simulink model "fm_gram"  (R2025b)
settings: Solver=ode2  StartTime=0.0  StopTime=5  FixedStep=1/400  RelTol=1e-3  EnableMultiTasking=on
PreLoadFcn:
  | stepsize_fm = evalin('base', get_param(bdroot, 'FixedStep'));
undefined symbols (not defined in the file or in its folder): Earth, F, Light, magnitude, MIL, propulsion, servo, vehicle, WGS84
libraries: slrealtimeutilitieslib x4, aerolibwind2 x2, sharedtransform x1, aerolib6dof2 x1, aerolibatmos2 x1, aerolibobsolete x1, slrealtimeiplib x1
settings Model: Creator=ac112430  LastModifiedBy=ac124458
settings SolverCC: AlgebraicLoopSolver=LineSearch
settings DataIOCC: ReturnWorkspaceOutputs=off
settings OptimizationCC: LifeSpan=inf
settings DebuggingCC: UnconnectedInputMsg=warning  UnconnectedOutputMsg=warning  UnconnectedLineMsg=warning  SFUnexpectedBacktrackingDiag=warning  SFNoUnconditionalDefaultTransitionDiag=warning  SFExecutionAtInitializationDiag=none  ArithmeticOperatorsInVariantConditions=warning
settings ModelReferenceCC: EnableRefExpFcnMdlSchedulingChecks=on
settings SFSimCC: SimUseLocalCustomCode=off  CustomCodeUndefinedFunction=UseInterfaceOnly
settings RTWCC: RTWUseLocalCustomCode=off  GPUComputeCapability=3.5
settings CodeAppCC: StateflowObjectComments=on
settings GRTTargetCC: TargetLangStandard=C89/C90 (ANSI)
settings ConfigComp: CovMetricSettings=dw  CovSaveCumulativeToWorkspaceVar=on  CovSaveSingleToWorkspaceVar=on  CovExternalEMLEnable=off

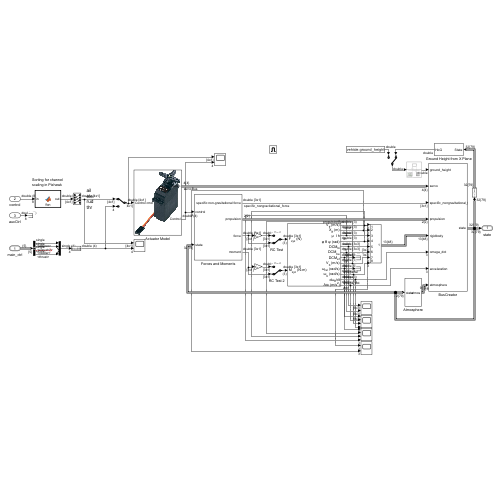
[thumbnail: Simulink's stored preview of the top-level diagram]
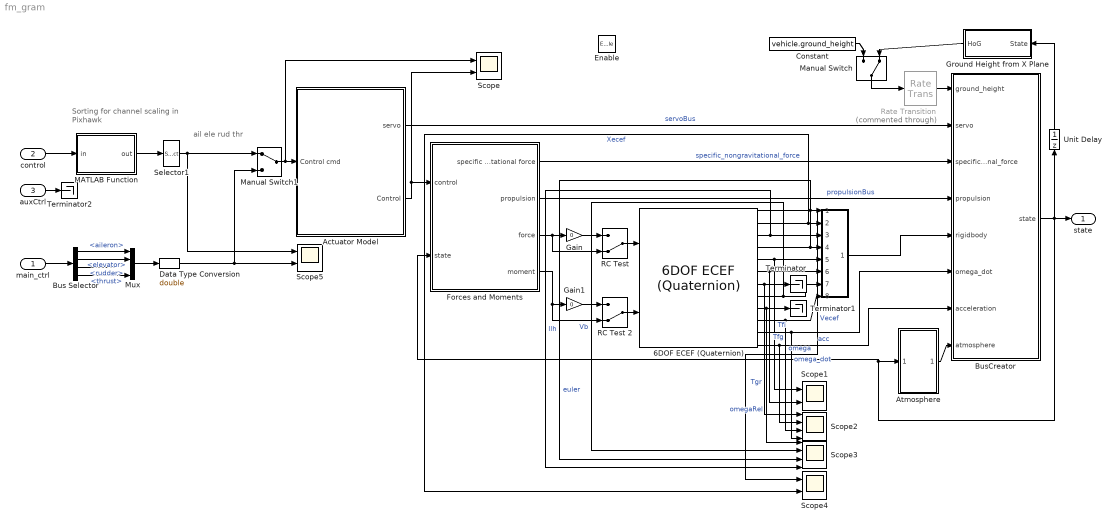
== system fm_gram ==
  note: ail
      | ele
      | rud
      | thr
  note: Sorting for channel
      | scaling in Pixhawk
  main_ctrl : Inport  OutDataTypeStr=Bus: main_ctrl_axes_bus  PortDimensions=1
  control : Inport  Port=2  PortDimensions=8
  auxCtrl : Inport  Port=3  PortDimensions=8
  Enable : EnablePort  PropagateVarSize=During execution
  " " : Subsystem
  6DOF ECEF (Quaternion) : aerolib6dof2/6DOF ECEF (Quaternion)  units=Metric (MKS)  mtype=Fixed  xg_0=vehicle.pos0  Vm_0=vehicle.vel0  eul_0=vehicle.ori0  pm_0=vehicle.omega0  mass_0=vehicle.m  mass_e=0.5  mass_f=2.0  inertia=vehicle.J  inertia_e=eye(3)  inertia_f=2*eye(3)  vre_flag=on  abi_flag=off  ptype=Earth (WGS84)  R=6378137  F=1/298.257223563  w_E=7292115e-11  angle_in=Internal  LPM0=0  quat_statename=''  pm_statename=''  Vm_statename=''  posfixedframe_statename=''  posinertial_statename=''  LPM_statename=''  mass_statename=''
  Actuator Model : Subsystem
      mask Display: image('figures\servo.jpg');
  Atmosphere : Subsystem
  Bus Selector : BusSelector  OutputSignals=aileron,elevator,rudder,thrust
  BusCreator : Subsystem
  Constant : Constant  Value=vehicle.ground_height  SampleTime=stepsize_fm
  Data Type Conversion : DataTypeConversion  OutDataTypeStr=double  SaturateOnIntegerOverflow=off  RndMeth=Floor
  Forces and Moments : Subsystem
  Gain : Gain  Gain=0
  Gain1 : Gain  Gain=0
  Ground Height from X Plane : Subsystem
  MATLAB Function : MATLAB Function  TreatAsAtomicUnit=on
  Manual Switch : ManualSwitch  CurrentSetting=0
  Manual Switch1 : ManualSwitch
  Mux : Mux
  RC Test : ManualSwitch  CurrentSetting=0
  RC Test 2 : ManualSwitch  CurrentSetting=0
  Rate Transition : RateTransition  Commented=through
  Scope{,1,4..5} (4 alike) : Scope  NumInputPorts=2
      Scope settings: ActiveDisplayYMinimum=-1.25  ActiveDisplayYMaximum=1.25
      Scope1 settings: ActiveDisplayYMinimum=-1  ActiveDisplayYMaximum=1  DataLoggingVariableName=ScopeData6
      Scope4 settings: ActiveDisplayYMinimum=-1.2221205757551141  ActiveDisplayYMaximum=1.2469022861950132  DataLoggingVariableName=ScopeData9
      Scope5 settings: ActiveDisplayYMinimum=-1.2414850783724674  ActiveDisplayYMaximum=1.2585150520126931
  Scope2 : Scope  NumInputPorts=4
      settings: ActiveDisplayYMinimum=-1  ActiveDisplayYMaximum=1  DataLoggingVariableName=ScopeData7
  Scope3 : Scope  NumInputPorts=4
      settings: ActiveDisplayYMinimum=-21.853179685501779  ActiveDisplayYMaximum=14.273381039110083  DataLoggingVariableName=ScopeData8
  Selector1 : Selector  InputPortWidth=4  IndexOptions=Index vector (dialog)  Indices=[2 3 4 1]  OutputSizes=1  RuntimeRangeChecks=on
  Terminator : Terminator
  Terminator1 : Terminator
  Terminator2 : Terminator
  Unit Delay : UnitDelay  SampleTime=-1  HasFrameUpgradeWarning=on
  state : Outport  OutDataTypeStr=Bus: fmBus  VectorParamsAs1DForOutWhenUnconnected=off
  wires:
  Forces and Moments/1(specific non-gravitational force) -> BusCreator/3(specific_nongravitational_force)  "specific_nongravitational_force"
  6DOF ECEF (Quaternion)/3 -> Scope3/4, " "/3(In3)  "llh"
  6DOF ECEF (Quaternion)/6 -> Scope1/2, " "/6(In6)  "Tfg"
  6DOF ECEF (Quaternion)/5 -> Scope1/1, " "/5(In5)  "Tfi"
  6DOF ECEF (Quaternion)/2 -> Scope4/2, " "/2(In2)  "Xecef"
  6DOF ECEF (Quaternion)/1 -> Scope4/1, " "/1(In1)  "Vecef"
  6DOF ECEF (Quaternion)/12 -> Scope2/2, BusCreator/7(acceleration)  "acc"
  6DOF ECEF (Quaternion)/8 -> Scope3/2, " "/7(In8)  "Vb"
  6DOF ECEF (Quaternion)/11 -> Scope2/4, BusCreator/6(omega_dot)  "omega_dot"
  Forces and Moments/2(propulsion) -> BusCreator/4(propulsion)  "propulsionBus"
  6DOF ECEF (Quaternion)/7 -> Scope2/1, Terminator/1  "Tgr"
  6DOF ECEF (Quaternion)/9 -> Terminator1/1, Scope3/1  "omegaRel"
  6DOF ECEF (Quaternion)/10 -> Scope2/3, " "/8(In10)  "omega"
  6DOF ECEF (Quaternion)/4 -> Scope3/3, " "/4(In4)  "euler"
  " "/1(Out1) -> BusCreator/5(rigidbody)
  Gain/1 -> RC Test/1
  Forces and Moments/3(force) -> RC Test/2, Gain/1
  Gain1/1 -> RC Test 2/1
  Forces and Moments/4(moment) -> RC Test 2/2, Gain1/1
  Actuator Model/2(Control) -> Scope/2, Forces and Moments/1(control)
  MATLAB Function/1(out) -> Selector1/1
  Actuator Model/1(servo) -> BusCreator/2(servo)  "servoBus"
  Ground Height from X Plane/1(HoG) -> Manual Switch/2
  Rate Transition/1 -> BusCreator/1(ground_height)
  control/1 -> MATLAB Function/1(in)
  Unit Delay/1 -> Ground Height from X Plane/1(State)
  auxCtrl/1 -> Terminator2/1
  Manual Switch/1 -> Rate Transition/1
  Constant/1 -> Manual Switch/1
  BusCreator/1(state) -> Forces and Moments/2(state), Atmosphere/1(state), Unit Delay/1, state/1
  Atmosphere/1(atmos) -> BusCreator/8(atmosphere)
  RC Test/1 -> 6DOF ECEF (Quaternion)/1
  RC Test 2/1 -> 6DOF ECEF (Quaternion)/2
  Mux/1 -> Data Type Conversion/1
  main_ctrl/1 -> Bus Selector/1
  Bus Selector/1 -> Mux/1  "<aileron>"
  Bus Selector/2 -> Mux/2  "<elevator>"
  Bus Selector/3 -> ?  "<rudder>"
  Bus Selector/4 -> Mux/4  "<thrust>"
  Selector1/1 -> Scope5/1, Manual Switch1/1
  Data Type Conversion/1 -> Manual Switch1/2, Scope5/2
  Manual Switch1/1 -> Scope/1, Actuator Model/1(Control cmd)

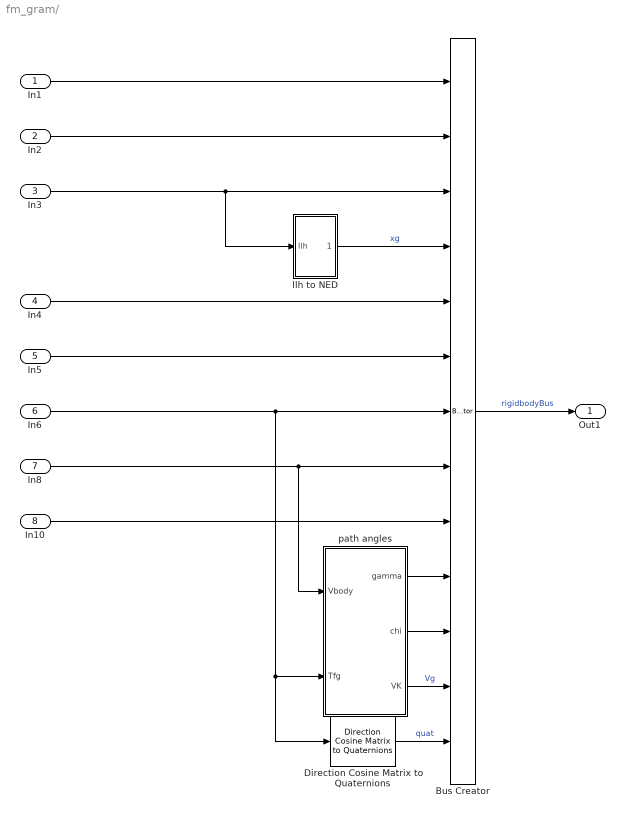
== system fm_gram/  ==
  In1 : Inport
  In2 : Inport  Port=2
  In3 : Inport  Port=3
  In4 : Inport  Port=4
  In5 : Inport  Port=5
  In6 : Inport  Port=6
  In8 : Inport  Port=7
  In10 : Inport  Port=8
  Bus Creator : BusCreator  Inputs=13  OutDataTypeStr=Bus: rigidbodyBus
  Direction Cosine Matrix to Quaternions : sharedtransform/Direction Cosine Matrix  to Quaternions  aMode=aMode  action=None  tolerance=eps(2)
  llh to NED : Subsystem
  path angles : MATLAB Function  TreatAsAtomicUnit=on
  Out1 : Outport  VectorParamsAs1DForOutWhenUnconnected=off
  wires:
  In10/1 -> Bus Creator/9
  path angles/2(chi) -> Bus Creator/11
  path angles/1(gamma) -> Bus Creator/10
  Direction Cosine Matrix to Quaternions/1 -> Bus Creator/13  "quat"
  In1/1 -> Bus Creator/1
  path angles/3(VK) -> Bus Creator/12  "Vg"
  In3/1 -> llh to NED/1(llh), Bus Creator/3
  In2/1 -> Bus Creator/2
  Bus Creator/1 -> Out1/1  "rigidbodyBus"
  In4/1 -> Bus Creator/5
  In8/1 -> path angles/1(Vbody), Bus Creator/8
  In6/1 -> Bus Creator/7, path angles/2(Tfg), Direction Cosine Matrix to Quaternions/1
  In5/1 -> Bus Creator/6
  llh to NED/1(NED) -> Bus Creator/4  "xg"

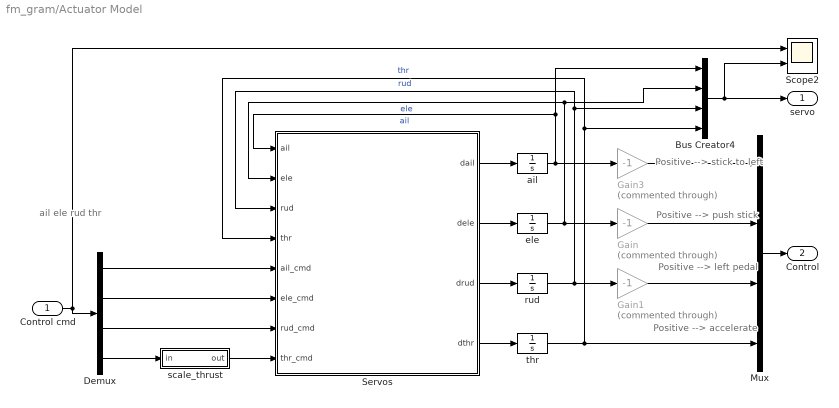
== system fm_gram/Actuator Model ==
  note: ail
      | ele
      | rud
      | thr
  note: Positive --> stick to left
  note: Positive --> left pedal
  note: Positive --> accelerate
  note: Positive --> push stick
  Control cmd : Inport
  Bus Creator4 : BusCreator  Inputs=4  OutDataTypeStr=Bus: servoBus
  Demux : Demux
  Gain : Gain  Commented=through  Gain=-1
  Gain1 : Gain  Commented=through  Gain=-1
  Gain3 : Gain  Commented=through  Gain=-1
  Mux : Mux
  Scope2 : Scope  NumInputPorts=2
      settings: ActiveDisplayYMinimum=-1.125  ActiveDisplayYMaximum=0.12499999999999997
  Servos : MATLAB Function  TreatAsAtomicUnit=on
  ail : Integrator  LimitOutput=on  UpperSaturationLimit=servo.ailLim(1)  LowerSaturationLimit=servo.ailLim(2)
  ele : Integrator  LimitOutput=on  UpperSaturationLimit=servo.eleLim(1)  LowerSaturationLimit=servo.eleLim(2)
  rud : Integrator  LimitOutput=on  UpperSaturationLimit=servo.rudLim(1)  LowerSaturationLimit=servo.rudLim(2)
  scale_thrust : MATLAB Function  TreatAsAtomicUnit=on
  thr : Integrator  LimitOutput=on  UpperSaturationLimit=servo.deltLim(1)  LowerSaturationLimit=servo.deltLim(2)
  servo : Outport  OutDataTypeStr=Bus: servoBus  VectorParamsAs1DForOutWhenUnconnected=off
  Control : Outport  Port=2
  wires:
  thr/1 -> Servos/4(thr), Bus Creator4/4, Mux/4  "thr"
  rud/1 -> Servos/3(rud), Bus Creator4/3, Gain1/1  "rud"
  ele/1 -> Bus Creator4/2, Servos/2(ele), Gain/1  "ele"
  Servos/4(dthr) -> thr/1
  Servos/1(dail) -> ail/1
  ail/1 -> Bus Creator4/1, Servos/1(ail), Gain3/1  "ail"
  Bus Creator4/1 -> Scope2/2, servo/1
  Control cmd/1 -> Scope2/1, Demux/1
  Mux/1 -> Control/1
  Demux/4 -> scale_thrust/1(in)
  Demux/3 -> Servos/7(rud_cmd)
  Demux/2 -> Servos/6(ele_cmd)
  Demux/1 -> Servos/5(ail_cmd)
  Servos/2(dele) -> ele/1
  Servos/3(drud) -> rud/1
  Gain/1 -> Mux/2
  Gain1/1 -> Mux/3
  Gain3/1 -> Mux/1
  scale_thrust/1(out) -> Servos/8(thr_cmd)

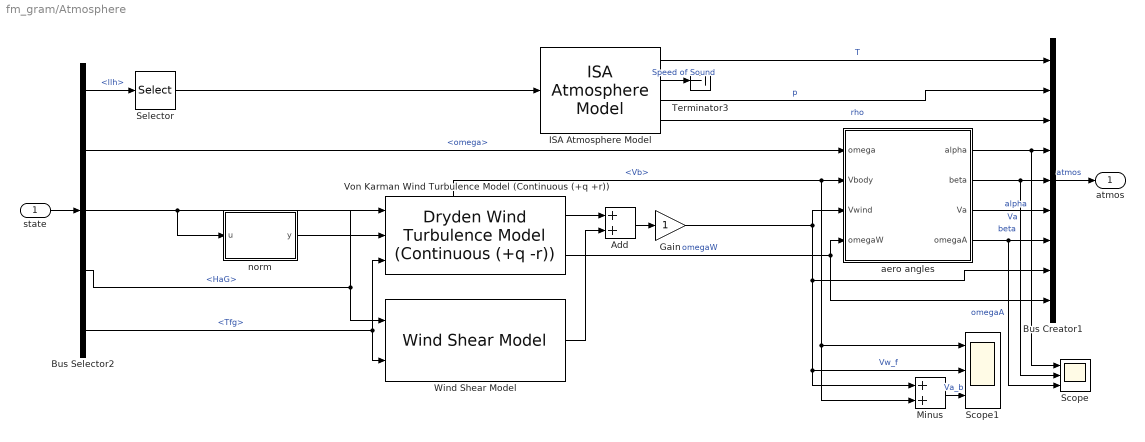
== system fm_gram/Atmosphere ==
  state : Inport
  Add : Sum
  Bus Creator1 : BusCreator  Inputs=9  OutDataTypeStr=Bus: atmosBus
  Bus Selector2 : BusSelector  OutputSignals=rigidbodyBus.llh,rigidbodyBus.omega,rigidbodyBus.Vb,utilityBus.HaG,rigidbodyBus.Tfg
  Gain : Gain
  ISA Atmosphere Model : aerolibatmos2/ISA Atmosphere Model  useExtended=off  action=None  custom=off  viscosityOut=off  g=9.80665  gamma=1.4  R=287.0531  L=0.0065  h_trop=11000  h_strat=20000  rho0=1.225  P0=101325  T0=288.15  h0=0  S=110.4  Tref=273.15  muref=1.716e-5
  Minus : Sum
  Scope : Scope  NumInputPorts=3
      settings: ActiveDisplayYMinimum=-2.50048  ActiveDisplayYMaximum=2.33546  DataLoggingVariableName=ScopeData3
  Scope1 : Scope  NumInputPorts=3
      settings: ActiveDisplayYMinimum=-12.555961798093179  ActiveDisplayYMaximum=23.617329088677021
  Selector : Selector  InputPortWidth=3  IndexOptions=Index vector (dialog)  Indices=3  OutputSizes=1
  Terminator3 : Terminator
  Von Karman Wind Turbulence Model (Continuous (+q +r)) : aerolibwind2/Dryden Wind Turbulence Model  (Continuous (+q -r))  units=Metric (MKS)  spec=MIL-F-8785C  model=Continuous Von Karman (+q +r)  W20=atmosphere.windStrength  Wdeg=atmosphere.windDir  TurbProb=10^-2 - Light  L_high=410  Wingspan=aerodynamic.b  ts=stepsize_fm  Seed=randi(20000,1,4)  T_on=off
  Wind Shear Model : aerolibwind2/Wind Shear Model  units=Metric (MKS)  phase=Other  W_20=atmosphere.windStrength  Wdeg=atmosphere.windDir
  aero angles : MATLAB Function  TreatAsAtomicUnit=on
  norm : MATLAB Function  TreatAsAtomicUnit=on
  atmos : Outport  OutDataTypeStr=Bus: atmosBus  VectorParamsAs1DForOutWhenUnconnected=off
  wires:
  Bus Creator1/1 -> atmos/1  "atmos"
  ISA Atmosphere Model/3 -> Bus Creator1/2  "p"
  ISA Atmosphere Model/1 -> Bus Creator1/1  "T"
  ISA Atmosphere Model/2 -> Terminator3/1  "Speed of Sound"
  Bus Selector2/1 -> Selector/1  "<llh>"
  Selector/1 -> ISA Atmosphere Model/1
  ISA Atmosphere Model/4 -> Bus Creator1/3  "rho"
  aero angles/1(alpha) -> Scope/1, Bus Creator1/4  "alpha"
  aero angles/2(beta) -> Scope/2, Bus Creator1/5  "beta"
  state/1 -> Bus Selector2/1
  Bus Selector2/2 -> aero angles/1(omega)  "<omega>"
  Wind Shear Model/1 -> Add/2
  norm/1(y) -> Von Karman Wind Turbulence Model (Continuous (+q +r))/2
  Von Karman Wind Turbulence Model (Continuous (+q +r))/1 -> Add/1
  Von Karman Wind Turbulence Model (Continuous (+q +r))/2 -> Bus Creator1/9, aero angles/4(omegaW)  "omegaW"
  Add/1 -> Gain/1
  Bus Selector2/5 -> Wind Shear Model/2, Von Karman Wind Turbulence Model (Continuous (+q +r))/3  "<Tfg>"
  aero angles/4(omegaA) -> Bus Creator1/7, Scope/3  "omegaA"
  Bus Selector2/4 -> Von Karman Wind Turbulence Model (Continuous (+q +r))/1, Wind Shear Model/1  "<HaG>"
  aero angles/3(Va) -> Bus Creator1/6  "Va"
  Minus/1 -> Scope1/3  "Va_b"
  Bus Selector2/3 -> Minus/2, Scope1/1, aero angles/2(Vbody), norm/1(u)  "<Vb>"
  Gain/1 -> Bus Creator1/8, Scope1/2, Minus/1, aero angles/3(Vwind)  "Vw_f"

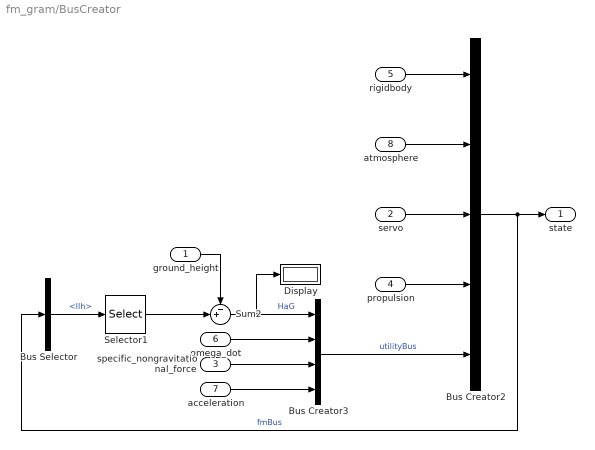
== system fm_gram/BusCreator ==
  ground_height : Inport
  servo : Inport  Port=2  OutDataTypeStr=Bus: servoBus
  specific_nongravitational_force : Inport  Port=3
  propulsion : Inport  Port=4  OutDataTypeStr=Bus: propulsionBus
  rigidbody : Inport  Port=5  OutDataTypeStr=Bus: rigidbodyBus
  omega_dot : Inport  Port=6
  acceleration : Inport  Port=7
  atmosphere : Inport  Port=8  OutDataTypeStr=Bus: atmosBus
  Bus Creator2 : BusCreator  Inputs=5  OutDataTypeStr=Bus: fmBus
  Bus Creator3 : BusCreator  Inputs=4  OutDataTypeStr=Bus: utilityBus
  Bus Selector : BusSelector  OutputSignals=rigidbodyBus.llh
  Display : Display
  Selector1 : Selector  InputPortWidth=3  IndexOptions=Index vector (dialog)  Indices=3  OutputSizes=1
  Sum2 : Sum  Inputs=-+|
  state : Outport  OutDataTypeStr=Bus: fmBus  VectorParamsAs1DForOutWhenUnconnected=off
  wires:
  Sum2/1 -> Display/1, Bus Creator3/1  "HaG"
  propulsion/1 -> Bus Creator2/4
  servo/1 -> Bus Creator2/3
  Bus Creator3/1 -> Bus Creator2/5  "utilityBus"
  Bus Creator2/1 -> state/1, Bus Selector/1  "fmBus"
  atmosphere/1 -> Bus Creator2/2
  Bus Selector/1 -> Selector1/1  "<llh>"
  rigidbody/1 -> Bus Creator2/1
  specific_nongravitational_force/1 -> Bus Creator3/3
  Selector1/1 -> Sum2/2
  ground_height/1 -> Sum2/1
  omega_dot/1 -> Bus Creator3/2
  acceleration/1 -> Bus Creator3/4

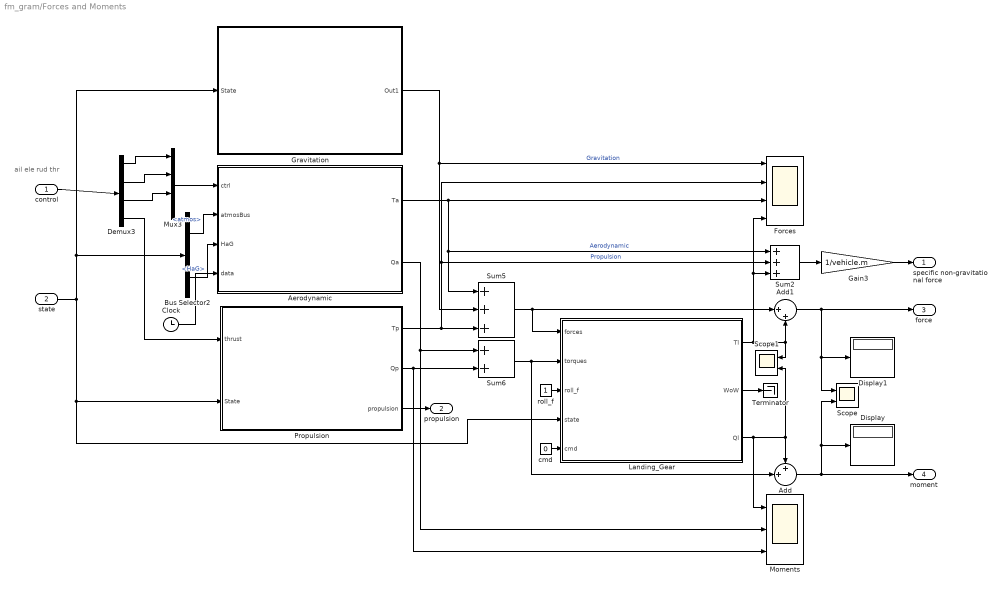
== system fm_gram/Forces and Moments ==
  note: ail
      | ele
      | rud
      | thr
  control : Inport
  state : Inport  Port=2
  Add : Sum  Inputs=++|
  Add1 : Sum  Inputs=|++
  Aerodynamic : MATLAB Function  TreatAsAtomicUnit=on
  Bus Selector2 : BusSelector  OutputSignals=atmos,utilityBus.HaG
  Clock : Clock
  Demux3 : Demux
  Display : Display
  Display1 : Display
  Forces : Scope  NumInputPorts=4
      settings: ActiveDisplayYMinimum=-8.4836089188338661  ActiveDisplayYMaximum=44.535465531132829
  Gain3 : Gain  Gain=1/vehicle.m
  Gravitation : Subsystem
      mask Display: image('figures\gravitation.jpg');
  Landing_Gear : Subsystem
      mask Display: image('C:\Workspace\funcub-xl\figures\LG.jpg'); % Use "Edit Image" on toolstrip to change.
  Moments : Scope  NumInputPorts=3
      settings: ActiveDisplayYMinimum=-12.453646898269653  ActiveDisplayYMaximum=7.4078247547149658  DataLoggingVariableName=ScopeData2
  Mux3 : Mux
  Propulsion : Subsystem
      mask Display: image('figures\propulsion.jpg');
  Scope : Scope  NumInputPorts=2
      settings: ActiveDisplayYMinimum=-87.1188785359822  ActiveDisplayYMaximum=56.206165438850242
  Scope1 : Scope  NumInputPorts=2
      settings: ActiveDisplayYMinimum=-7.91236  ActiveDisplayYMaximum=9.60283
  Sum2 : Sum  Inputs=+++
  Sum5 : Sum  Inputs=+++
  Sum6 : Sum
  Terminator : Terminator
  cmd : Constant  Value=0
  roll_f : Constant
  specific non-gravitational force : Outport  VectorParamsAs1DForOutWhenUnconnected=off
  propulsion : Outport  Port=2  VectorParamsAs1DForOutWhenUnconnected=off
  force : Outport  Port=3  VectorParamsAs1DForOutWhenUnconnected=off
  moment : Outport  Port=4  VectorParamsAs1DForOutWhenUnconnected=off
  wires:
  Gain3/1 -> specific non-gravitational force/1
  Demux3/4 -> Propulsion/1(thrust)
  control/1 -> Demux3/1
  Propulsion/3(propulsion) -> propulsion/1
  Gravitation/1(Out1) -> Sum5/2, Forces/1  "Gravitation"
  Demux3/2 -> Mux3/2
  Demux3/3 -> Mux3/3
  Demux3/1 -> Mux3/1
  Aerodynamic/1(Ta) -> Forces/3, Sum5/1, Sum2/1  "Aerodynamic"
  Propulsion/1(Tp) -> Forces/2, Sum2/2, Sum5/3  "Propulsion"
  roll_f/1 -> Landing_Gear/3(roll_f)
  Landing_Gear/1(Tl) -> Add1/2, Scope1/1, Forces/4, Sum2/3
  Landing_Gear/3(Ql) -> Moments/1, Scope1/2, Add/1
  state/1 -> Landing_Gear/4(state), Propulsion/2(State), Gravitation/1(State), Bus Selector2/1
  Bus Selector2/1 -> Aerodynamic/2(atmosBus)  "<atmos>"
  Bus Selector2/2 -> Aerodynamic/3(HaG)  "<HaG>"
  Mux3/1 -> Aerodynamic/1(ctrl)
  Add1/1 -> Display1/1, Scope/1, force/1
  Add/1 -> moment/1, Scope/2, Display/1
  Sum2/1 -> Gain3/1
  Propulsion/2(Qp) -> Moments/3, Sum6/2
  Aerodynamic/2(Qa) -> Moments/2, Sum6/1
  Sum5/1 -> Add1/1, Landing_Gear/1(forces)
  Sum6/1 -> Add/2, Landing_Gear/2(torques)
  Landing_Gear/2(WoW) -> Terminator/1
  Clock/1 -> Aerodynamic/4(data)
  cmd/1 -> Landing_Gear/5(cmd)

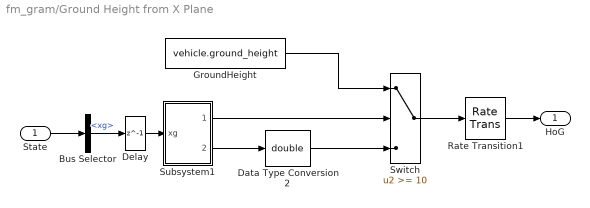
== system fm_gram/Ground Height from X Plane ==
  State : Inport
  Bus Selector : BusSelector  OutputSignals=rigidbodyBus.xg
  Data Type Conversion2 : DataTypeConversion  OutDataTypeStr=double  SaturateOnIntegerOverflow=off  RndMeth=Floor
  Delay : Delay  DelayLength=1
  GroundHeight : Constant  Value=vehicle.ground_height  SampleTime=-1
  Rate Transition1 : RateTransition  OutPortSampleTime=stepsize_fm
  Subsystem1 : Subsystem
  Switch : Switch  Threshold=10  SaturateOnIntegerOverflow=off  InputSameDT=off
  HoG : Outport  VectorParamsAs1DForOutWhenUnconnected=off
  wires:
  Subsystem1/2(Out1) -> Data Type Conversion2/1
  Rate Transition1/1 -> HoG/1
  Switch/1 -> Rate Transition1/1
  GroundHeight/1 -> Switch/1
  Data Type Conversion2/1 -> Switch/3
  Subsystem1/1(Out2) -> Switch/2
  Delay/1 -> Subsystem1/1(xg)
  State/1 -> Bus Selector/1
  Bus Selector/1 -> Delay/1  "<xg>"

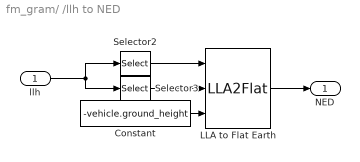
== system fm_gram/ /llh to NED ==
  llh : Inport
  Constant : Constant  Value=-vehicle.ground_height
  LLA to Flat Earth : LLA2Flat  R=6378137  LL0=vehicle.pos0(1:2)
  Selector2 : Selector  InputPortWidth=3  IndexOptions=Index vector (dialog)  Indices=1:2  OutputSizes=1
  Selector3 : Selector  InputPortWidth=3  IndexOptions=Index vector (dialog)  Indices=3  OutputSizes=1
  NED : Outport  VectorParamsAs1DForOutWhenUnconnected=off
  wires:
  LLA to Flat Earth/1 -> NED/1
  llh/1 -> Selector3/1, Selector2/1
  Constant/1 -> LLA to Flat Earth/3
  Selector2/1 -> LLA to Flat Earth/1
  Selector3/1 -> LLA to Flat Earth/2

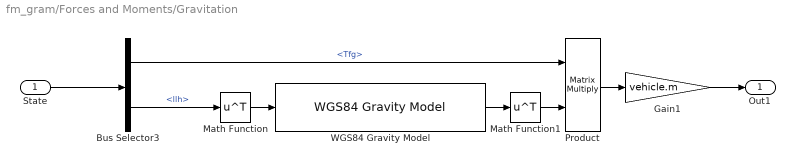
== system fm_gram/Forces and Moments/Gravitation ==
  State : Inport  OutDataTypeStr=Bus: fmBus
  Bus Selector3 : BusSelector  OutputSignals=rigidbodyBus.Tfg,rigidbodyBus.llh
  Gain1 : Gain  Gain=vehicle.m
  Math Function : Math  Operator=transpose  SignedPower=on
  Math Function1 : Math  Operator=transpose  SignedPower=on
  Product : Product  Multiplication=Matrix(*)
  "WGS84 Gravity Model " : aerolibobsolete/WGS84 Gravity Model   model=WGS84 Taylor Series  units=Metric (MKS)  no_atmos=on  precessing=on  jd_loc=off  month=October  day=10  year=2004  no_centrifugal=on  action=Warning
  Out1 : Outport
  wires:
  Math Function/1 -> "WGS84 Gravity Model "/1
  "WGS84 Gravity Model "/1 -> Math Function1/1
  Product/1 -> Gain1/1
  Gain1/1 -> Out1/1
  Math Function1/1 -> Product/2
  Bus Selector3/1 -> Product/1  "<Tfg>"
  Bus Selector3/2 -> Math Function/1  "<llh>"
  State/1 -> Bus Selector3/1

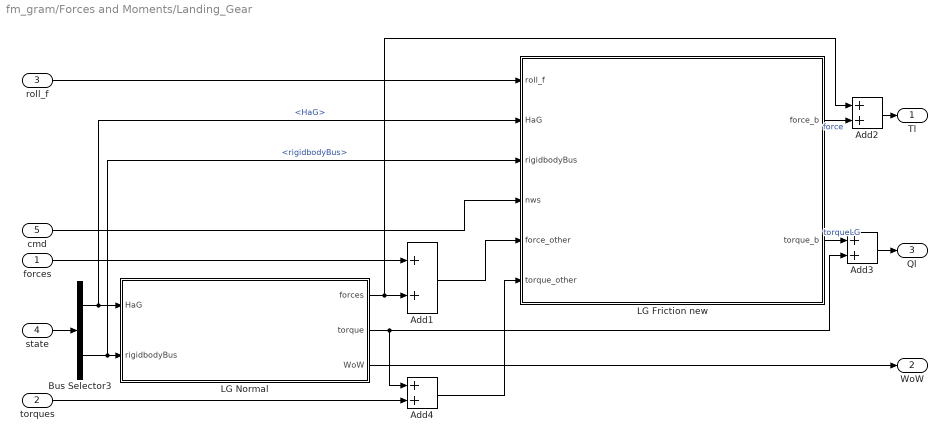
== system fm_gram/Forces and Moments/Landing_Gear ==
  forces : Inport
  torques : Inport  Port=2
  roll_f : Inport  Port=3
  state : Inport  Port=4  OutDataTypeStr=Bus: fmBus
  cmd : Inport  Port=5
  Add1 : Sum
  Add2 : Sum  OutDataTypeStr=single  AccumDataTypeStr=single
  Add3 : Sum  OutDataTypeStr=single  AccumDataTypeStr=single
  Add4 : Sum
  Bus Selector3 : BusSelector  OutputSignals=utilityBus.HaG,rigidbodyBus
  LG Friction new : MATLAB Function  TreatAsAtomicUnit=on
  LG Normal : MATLAB Function  TreatAsAtomicUnit=on
  Tl : Outport
  WoW : Outport  Port=2  OutDataTypeStr=boolean
  Ql : Outport  Port=3
  wires:
  Bus Selector3/1 -> LG Friction new/2(HaG), LG Normal/1(HaG)  "<HaG>"
  Bus Selector3/2 -> LG Friction new/3(rigidbodyBus), LG Normal/2(rigidbodyBus)  "<rigidbodyBus>"
  LG Normal/3(WoW) -> WoW/1
  roll_f/1 -> LG Friction new/1(roll_f)
  Add4/1 -> LG Friction new/6(torque_other)
  Add2/1 -> Tl/1
  Add3/1 -> Ql/1
  LG Friction new/2(torque_b) -> Add3/1  "torqueLG"
  LG Friction new/1(force_b) -> Add2/2  "force"
  Add1/1 -> LG Friction new/5(force_other)
  LG Normal/1(forces) -> Add2/1, Add1/2
  LG Normal/2(torque) -> Add4/1, Add3/2
  forces/1 -> Add1/1
  torques/1 -> Add4/2
  cmd/1 -> LG Friction new/4(nws)
  state/1 -> Bus Selector3/1

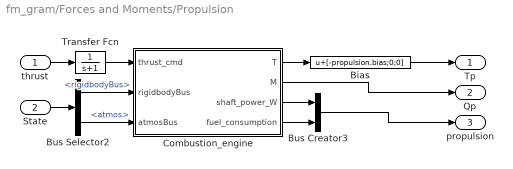
== system fm_gram/Forces and Moments/Propulsion ==
  thrust : Inport
  State : Inport  Port=2  OutDataTypeStr=Bus: fmBus
  Bias : Bias  Bias=[-propulsion.bias;0;0]  SaturateOnIntegerOverflow=off
  Bus Creator3 : BusCreator  Inputs=2  OutDataTypeStr=Bus: propulsionBus
  Bus Selector2 : BusSelector  OutputSignals=rigidbodyBus,atmos
  Combustion_engine : MATLAB Function  TreatAsAtomicUnit=on
  Transfer Fcn : TransferFcn  Denominator=[1 1]
  Tp : Outport
  Qp : Outport  Port=2
  propulsion : Outport  Port=3  VectorParamsAs1DForOutWhenUnconnected=off
  wires:
  Bus Creator3/1 -> propulsion/1
  State/1 -> Bus Selector2/1
  Transfer Fcn/1 -> Combustion_engine/1(thrust_cmd)
  Combustion_engine/1(T) -> Bias/1
  Bus Selector2/2 -> Combustion_engine/3(atmosBus)  "<atmos>"
  Bus Selector2/1 -> Combustion_engine/2(rigidbodyBus)  "<rigidbodyBus>"
  thrust/1 -> Transfer Fcn/1
  Bias/1 -> Tp/1
  Combustion_engine/2(M) -> Qp/1
  Combustion_engine/3(shaft_power_W) -> Bus Creator3/1
  Combustion_engine/4(fuel_consumption) -> Bus Creator3/2

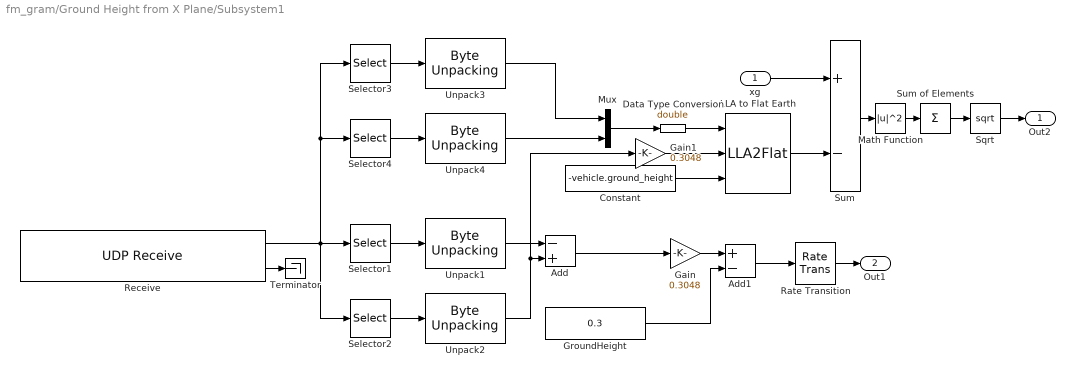
== system fm_gram/Ground Height from X Plane/Subsystem1 ==
  xg : Inport
  Add : Sum  Inputs=-+
  Add1 : Sum  Inputs=+-
  Constant : Constant  Value=-vehicle.ground_height
  Data Type Conversion : DataTypeConversion  OutDataTypeStr=double  SaturateOnIntegerOverflow=off  RndMeth=Floor
  Gain : Gain  Gain=0.3048
  Gain1 : Gain  Gain=0.3048  OutDataTypeStr=double
  GroundHeight : Constant  Value=0.3  SampleTime=-1
  LLA to Flat Earth : LLA2Flat  R=6378137  LL0=vehicle.pos0(1:2)
  Math Function : Math  Operator=magnitude^2  SignedPower=on
  Mux : Mux  Inputs=2
  Rate Transition : RateTransition
  Receive : slrealtimeiplib/UDP Receive  useHostTargetConn=on  ipAddress=10.10.10.15  localPort=12345  rcvWidth=41  rcvFmAny=off  fmAddress=129.69.124.62  sampleTime=stepsize_fm  enableMessage=off  maxPackets=1
  Selector1 : Selector  InputPortWidth=41  IndexOptions=Index vector (dialog)  Indices=[22:25]  OutputSizes=1
  Selector2 : Selector  InputPortWidth=41  IndexOptions=Index vector (dialog)  Indices=[18:21]  OutputSizes=1
  Selector3 : Selector  InputPortWidth=41  IndexOptions=Index vector (dialog)  Indices=[10:13]  OutputSizes=1
  Selector4 : Selector  InputPortWidth=41  IndexOptions=Index vector (dialog)  Indices=[14:17]  OutputSizes=1
  Sqrt : Sqrt
  Sum : Sum  Inputs=+-
  Sum of Elements : Sum  Inputs=+
  Terminator : Terminator
  Unpack{1..4} (4 alike) : slrealtimeutilitieslib/Byte Unpacking  MaskUnpackedDataTypes={'single'}  MaskUnpackedDataSizes={[1]}  MaskAlignment=1
  Out2 : Outport  VectorParamsAs1DForOutWhenUnconnected=off
  Out1 : Outport  Port=2  VectorParamsAs1DForOutWhenUnconnected=off
  wires:
  Gain/1 -> Add1/1
  Add1/1 -> Rate Transition/1
  GroundHeight/1 -> Add1/2
  Selector1/1 -> Unpack1/1
  Receive/2 -> Terminator/1
  Selector2/1 -> Unpack2/1
  Unpack1/1 -> Add/1
  Unpack2/1 -> Gain1/1, Add/2
  Add/1 -> Gain/1
  Rate Transition/1 -> Out1/1
  Selector3/1 -> Unpack3/1
  Selector4/1 -> Unpack4/1
  Receive/1 -> Selector3/1, Selector4/1, Selector2/1, Selector1/1
  Unpack3/1 -> Mux/1
  Unpack4/1 -> Mux/2
  Constant/1 -> LLA to Flat Earth/3
  Mux/1 -> Data Type Conversion/1
  LLA to Flat Earth/1 -> Sum/2
  xg/1 -> Sum/1
  Gain1/1 -> LLA to Flat Earth/2
  Sum/1 -> Math Function/1
  Math Function/1 -> Sum of Elements/1
  Sum of Elements/1 -> Sqrt/1
  Sqrt/1 -> Out2/1
  Data Type Conversion/1 -> LLA to Flat Earth/1

== matlab function fm_gram/Forces and Moments/Landing_Gear/LG Normal ==
  data: HaG input; rigidbodyBus input; forces output; torque output; WoW output; vehicle parameter
function [forces,torque,WoW] = LG_normal_forces(HaG,rigidbodyBus,vehicle)
euler = rigidbodyBus.euler;
omega = rigidbodyBus.omega;
Vg    = rigidbodyBus.Vg;
WoW   = [false false]';
CG    = vehicle.cg;
gear  = vehicle.gear;

%% gear compression and velocities
pos_right_cg = gear.right_pos - CG;
pos_left_cg  = gear.left_pos - CG;
pos_aux_cg  = gear.aux_pos - CG;

Tfg = angle2rotation(euler(1),euler(2),euler(3));                           % Tfg => transformation matrix geodetic to body
Tgf = Tfg';                                                                 % Tgf => transformation matrix geodetic body to geodetic

pos_right_g = Tgf * pos_right_cg;                                           % pos_right_g   => position of right gear in geodetic system
pos_left_g  = Tgf * pos_left_cg;                                            % pos_left_g    => position of left gear in geodetic system
pos_aux_g  = Tgf * pos_aux_cg;                                            % pos_aux_g    => position of nose/tail gear in geodetic system

compression_right = max(0,pos_right_g(3) - HaG);                            
compression_left  = max(0,pos_left_g(3)  - HaG);
compression_aux  = max(0,pos_aux_g(3)  - HaG);
WoW(1) = compression_right > 0;
WoW(2) = compression_left  > 0;

omegaG = Tgf * omega;
Vg_right = Vg + cross(omegaG, pos_right_g);
Vg_left  = Vg + cross(omegaG, pos_left_g);
Vg_aux  = Vg + cross(omegaG, pos_aux_g);

%% compression and dampening forces
comp_force_right = -gear.main_stiff * compression_right * [0; 0; 1];
damp_force_right = -gear.main_damp  * Vg_right(3) * (compression_right > 0) * [0; 0; 1];

comp_force_left  = -gear.main_stiff * compression_left * [0; 0; 1];
damp_force_left  = -gear.main_damp  * Vg_left(3) * (compression_left > 0) * [0; 0; 1];

comp_force_aux  = -gear.aux_stiff * compression_aux * [0; 0; 1];
damp_force_aux  = -gear.aux_damp  * Vg_aux(3) * (compression_aux > 0) * [0; 0; 1];

forces_right = comp_force_right + damp_force_right;
forces_left  = comp_force_left  + damp_force_left;
forces_aux  = comp_force_aux  + damp_force_aux;

%% resulting forces and torques, geo to body
% torque due to gear positions
torque_right = cross(pos_right_g, forces_right);
torque_left  = cross(pos_left_g,  forces_left);
torque_aux  = cross(pos_aux_g,  forces_aux);

% total forces and moments (inertial)
forces_g = forces_right + forces_left + forces_aux;
torque_g = torque_right + torque_left + torque_aux;

% transformation to body frame
forces = Tfg * forces_g;
torque = Tfg * torque_g;

end

function dcm = angle2rotation(phi,theta,psi)
t1 = [1 0 0;0 cos(phi) sin(phi);0 -sin(phi) cos(phi)];
t2 = [cos(theta) 0 -sin(theta);0 1 0;sin(theta) 0 cos(theta)];
t3 = [cos(psi) sin(psi) 0;-sin(psi) cos(psi) 0;0 0 1];
dcm = t1*t2*t3;
end

== matlab function fm_gram/Atmosphere/aero angles ==
  data: omega input size=3; Vbody input; Vwind input; omegaW input size=3; alpha output; beta output; Va output; omegaA output size=3
function [alpha,beta,Va,omegaA] = calcAeroAngles(omega,Vbody,Vwind,omegaW)
bVa = Vbody+Vwind;
if abs(bVa(1))>1
    alpha = atan2(bVa(3),bVa(1));
else
    alpha = 0;
end
if norm(bVa)>1
    beta  = asin(bVa(2)/norm(bVa));
else
    beta = 0;
end
Va    = norm(bVa);
omegaA = omega + omegaW;

== matlab function fm_gram/Atmosphere/norm ==
  data: u input; y output
function y = norm(u)
%#codegen

y = norm(u);
if y < 1
    y = 1;
end

== matlab function fm_gram/ /path angles ==
  data: Vbody input; Tfg input; gamma output; chi output; VK output
function [gamma,chi,VK] = calcPathAngles(Vbody,Tfg)
VK = Tfg'*Vbody;
if norm(VK)>0.1
    gamma = -asin(VK(3)/norm(VK));
else
    gamma = 0;
end
chi   = atan2(VK(2),VK(1));

== matlab function fm_gram/Actuator Model/scale_thrust ==
  data: in input; out output
function out = fcn(in)

out = max(0,min(1,(in+1)/2)); %scale thrust from [-1,1] to [0,1]

== matlab function fm_gram/MATLAB Function ==
  data: in input; out output
function out = fcn(in)
out = zeros(4,1);

out(1) = in(1); %thr
out(2) = 3/2*(in(5)-in(6))/2; %ail
out(3) = 3/2*(in(5)+in(6))/2; %ele
out(4) = 0; %rud

== matlab function fm_gram/Forces and Moments/Propulsion/Combustion_engine ==
  data: thrust_cmd input; T output; rigidbodyBus input; atmosBus input; propulsion parameter; M output; shaft_power_W output; fuel_consumption output
function [T,M,shaft_power_W,fuel_consumption] = fcn(thrust_cmd,rigidbodyBus,atmosBus,propulsion)
T = zeros(3,1);
M = zeros(3,1);

% Velocities
Vzinf = (atmosBus.Va*cos(atmosBus.alpha))*cos(atmosBus.beta); % perpendicular to propeller disk

% Thrust forces and moments
thrust_cmd = min(max(thrust_cmd,0),1);
thrust_per = 0.4258*thrust_cmd^4 - 0.4724*thrust_cmd^3 - 1.1373*thrust_cmd^2 + 1.9888*thrust_cmd; %from "New Thrust Model.xlsx"

Vzinf_kts = Vzinf*3.6/1.852;
shaft_power_W = thrust_per*propulsion.power_max;
shaft_power_hp = shaft_power_W / 745.699872;
% from Snorri Gudmundsson "General Aviation Aircraft Design Second Edition"
% p.633
% Calculation of following parameters for prop efficiency in "New Thrust Model.xlsx"
A1 = 0.009684897;
A2 = -1.65106E-05;
A3 = -1.55903E-07;
A4 = 4.74652E-10;

thrust_lbf = 325.9*(A1+A2*Vzinf_kts+A3*Vzinf_kts^2+A4*Vzinf_kts^3)*shaft_power_hp;
thrust = thrust_lbf*4.44822162;
% Calculation of following parameters in "Standschub Analyse.xlsx"
fuel_consumption = 7e-14*shaft_power_W^3 - 7e-9*shaft_power_W^2 + 0.0032*shaft_power_W + 15.95;

% force effect due to aerodynamic angles
T(1) = thrust * cos(propulsion.inci);
T(2) = 0;
T(3) = thrust * sin(propulsion.inci);

% moment effect due to engine position
M(1) =  thrust * sin(propulsion.inci) * propulsion.r(2);
M(2) =  thrust * (cos(propulsion.inci)* propulsion.r(3)- sin(propulsion.inci)*propulsion.r(1));
M(3) = -thrust * cos(propulsion.inci) * propulsion.r(2);

end

== matlab function fm_gram/Forces and Moments/Aerodynamic ==
  data: ctrl input; atmosBus input; HaG input; Ta output; Qa output; aerodynamic parameter; data input
function [Ta,Qa]= aerodynamic(ctrl,atmosBus,HaG,aerodynamic,data)
MAX_FLAP_DEG = deg2rad(30); %maximum flap angle setting in XFLR5 model

ail = ctrl(1);
ele = ctrl(2);
rud  = ctrl(3);
flp  = ctrl(4);

omegaA = atmosBus.omegaA;
Va    = atmosBus.Va;
rho   = atmosBus.rho;
alpha = atmosBus.alpha;
beta  = atmosBus.beta;

Tfs = stabilityToBody(alpha);
pdyn = 0.5*rho*Va^2;

if Va > 1
    pstar = omegaA(1)*aerodynamic.b/(2*Va);
    qstar = omegaA(2)*aerodynamic.chord/(2*Va);
    rstar = omegaA(3)*aerodynamic.b/(2*Va);
else
    Valim = 1;
    pstar = omegaA(1)*aerodynamic.b/(2*Valim);
    qstar = omegaA(2)*aerodynamic.chord/(2*Valim);
    rstar = omegaA(3)*aerodynamic.b/(2*Valim);
end

%% aero_struct_old == 1, only flaps0
VaLim = lim(Va,aerodynamic.derivatives.vBounds);

% Pitch Rate
CDq  = interp1(aerodynamic.derivatives.VInf,aerodynamic.derivatives.CDq,VaLim);
CLq  = interp1(aerodynamic.derivatives.VInf,aerodynamic.derivatives.CLq,VaLim);
Cmq  = interp1(aerodynamic.derivatives.VInf,aerodynamic.derivatives.Cmq,VaLim);

% Roll Rate
CYp  = interp1(aerodynamic.derivatives.VInf,aerodynamic.derivatives.CYp,VaLim);
Clp  = interp1(aerodynamic.derivatives.VInf,aerodynamic.derivatives.Clp,VaLim);
Cnp  = interp1(aerodynamic.derivatives.VInf,aerodynamic.derivatives.Cnp,VaLim);

% Yaw Rate
CYr  = interp1(aerodynamic.derivatives.VInf,aerodynamic.derivatives.CYr,VaLim);
Clr  = interp1(aerodynamic.derivatives.VInf,aerodynamic.derivatives.Clr,VaLim);
Cnr  = interp1(aerodynamic.derivatives.VInf,aerodynamic.derivatives.Cnr,VaLim);

% Elevator
CDele  = interp1(aerodynamic.derivatives.VInf,aerodynamic.derivatives.CDele,VaLim);
CLele  = interp1(aerodynamic.derivatives.VInf,aerodynamic.derivatives.CLele,VaLim);
Cmele  = interp1(aerodynamic.derivatives.VInf,aerodynamic.derivatives.Cmele,VaLim);

% Aileron
CYail  = aerodynamic.derivatives.CYail;
Clail  = aerodynamic.derivatives.Clail;
Cnail  = aerodynamic.derivatives.Cnail;

% Rudder
CYrud  = aerodynamic.derivatives.CYrud;
Clrud  = aerodynamic.derivatives.Clrud;
Cnrud  = aerodynamic.derivatives.Cnrud;

VaLim = lim(Va,aerodynamic.polar.vBounds);
alphaLim = lim(alpha,aerodynamic.polar.alphaBounds);
fbetaLim = lim(abs(beta),aerodynamic.polar.betaBounds);

% Polar
CD0 = interp3(aerodynamic.polar.beta,aerodynamic.polar.alpha,aerodynamic.polar.V,aerodynamic.polar.CD,fbetaLim,alphaLim,VaLim);
CY0 = sign(beta)*interp3(aerodynamic.polar.beta,aerodynamic.polar.alpha,aerodynamic.polar.V,aerodynamic.polar.CY,fbetaLim,alphaLim,VaLim);
CL0 = interp3(aerodynamic.polar.beta,aerodynamic.polar.alpha,aerodynamic.polar.V,aerodynamic.polar.CL,fbetaLim,alphaLim,VaLim);
Cl0 = sign(beta)*interp3(aerodynamic.polar.beta,aerodynamic.polar.alpha,aerodynamic.polar.V,aerodynamic.polar.Cl,fbetaLim,alphaLim,VaLim);
Cn0 = sign(beta)*interp3(aerodynamic.polar.beta,aerodynamic.polar.alpha,aerodynamic.polar.V,aerodynamic.polar.Cn,fbetaLim,alphaLim,VaLim);
[alphaGE,CL0,CD0] = groundEffect(alpha,CL0,CD0,HaG,aerodynamic.b,aerodynamic.chord,aerodynamic.alpha0);
alphaLimGE = lim(alphaGE,aerodynamic.polar.alphaBounds);
Cm0 = interp3(aerodynamic.polar.beta,aerodynamic.polar.alpha,aerodynamic.polar.V,aerodynamic.polar.Cm,fbetaLim,alphaLimGE,VaLim);

%% Aggregation
CD = CD0 + CDq*qstar + CDele*ele;% + CDflp*flp;
CL = CL0 + CLq*qstar + CLele*ele;% + CLflp*flp;
CY = CY0 + CYp*pstar + CYr*rstar + CYail*ail + CYrud*rud;
Cl = Cl0 + Clp*pstar + Clr*rstar + Clail*ail + Clrud*rud;
Cm = Cm0 + Cmq*qstar + Cmele*ele;
Cn = Cn0 + Cnp*pstar + Cnr*rstar + Cnail*ail + Cnrud*rud;

%Monitor
D_moni = [CD,CD0,CDq*qstar,CDele*ele];
L_moni = [CL,CL0,CLq*qstar,CLele*ele];

% Force and Torque in wind frame
aTa = [-CD;CY;-CL]*pdyn*aerodynamic.S;
aQa = [Cl*aerodynamic.b;Cm*aerodynamic.chord;Cn*aerodynamic.b]*pdyn*aerodynamic.S;

% Force and Torque in body frame
Ta = Tfs*aTa;
Qa = Tfs*aQa;

end

function [alpha,CL,CD] = groundEffect(alpha,CL,CD,HaG,b,c,alpha0)

%  b: Spannweite, t: Profiltiefe
t       = c/12;  % Profildicke, Schätzung!
e       = 0.8;   % Oswald
AR      = b/c;   % Streckung
CLalpha = liftSlope(AR,0,0); % Endliche ebene Platte, Pfeilung = 0

% Ground Effect Parameters
WaG    = [ 0, 0.1, 0.2, 0.3, 0.4, 0.5, 0.6, 0.7, 0.8, 0.9, 1.0, 1.1, 1.2, 1.3, 1.4, 1.5, 1.6, 1.7, 1.8, 1.9, 2.0];
AACOef = [ 0, 0.3, 0.5, 0.6, 0.68, 0.73, 0.77, 0.82, 0.855, 0.885,0.915, 0.93, 0.94, 0.965, 0.973, 0.98, 0.985, 0.99, 0.995, 1, 1];

Wing_hag = HaG/b;
Cord_hag = HaG/t;

if (Wing_hag < 0.01)
    Wing_hag = 0.01;
end

if (Wing_hag < 2)

    ind = sum(WaG < Wing_hag) + 1;

    sigma   = (1 - 1.32*Wing_hag)/(1.05 + 7.4*Wing_hag);
    if sigma < 0
        sigma = 0;
    end
    CD = CD - sigma*(CL^2)/(pi*AR*e); % Calculated with out of GE lift!

    AReff      = AR/interp1(WaG,AACOef,Wing_hag);
    CLalphaEff = liftSlope(AReff,0,0);
    dalpha0    = t/c*pi*(3.5655/Cord_hag - 0.1177/Cord_hag^2)/180.0;

    CL = CL-CLalpha*(alpha-alpha0)+CLalphaEff*(alpha - dalpha0 - alpha0);
    alpha = alpha - dalpha0;

end

end

function Cla = liftSlope(AR,lambda,Ma)
Cla0 = 2*pi; % Auftriebsanstieg Profil
Cla = Cla0*cos(lambda)/(sqrt(1-Ma^2*cos(lambda)^2+(Cla0*cos(lambda)/(pi*AR))^2)+Cla0*cos(lambda)/(pi*AR));
end

function t = stabilityToBody(alpha)
t = [cos(alpha) 0 -sin(alpha); 0 1 0; sin(alpha) 0 cos(alpha)];
end

function y = lim(y,bounds)
y = max(bounds(1),min(bounds(2),y));
end

function [CDq, CLq, Cmq, CYp, Clp, Cnp, CYr, Clr, Cnr,CDele, CLele, Cmele] = interpolateFlaps(valid_elements,VaLim,aerodynamic,column)
VInf = aerodynamic.derivatives.VInf(1:valid_elements,column);

% Pitch Rate
CDq  = interp1(VInf,aerodynamic.derivatives.CDq(1:valid_elements,column),VaLim);
CLq  = interp1(VInf,aerodynamic.derivatives.CLq(1:valid_elements,column),VaLim);
Cmq  = interp1(VInf,aerodynamic.derivatives.Cmq(1:valid_elements,column),VaLim);

% Roll Rate
CYp  = interp1(VInf,aerodynamic.derivatives.CYp(1:valid_elements,column),VaLim);
Clp  = interp1(VInf,aerodynamic.derivatives.Clp(1:valid_elements,column),VaLim);
Cnp  = interp1(VInf,aerodynamic.derivatives.Cnp(1:valid_elements,column),VaLim);

% Yaw Rate
CYr  = interp1(VInf,aerodynamic.derivatives.CYr(1:valid_elements,column),VaLim);
Clr  = interp1(VInf,aerodynamic.derivatives.Clr(1:valid_elements,column),VaLim);
Cnr  = interp1(VInf,aerodynamic.derivatives.Cnr(1:valid_elements,column),VaLim);

% Elevator
CDele  = interp1(VInf,aerodynamic.derivatives.CDele(1:valid_elements,column),VaLim);
CLele  = interp1(VInf,aerodynamic.derivatives.CLele(1:valid_elements,column),VaLim);
Cmele  = interp1(VInf,aerodynamic.derivatives.Cmele(1:valid_elements,column),VaLim);
end

== matlab function fm_gram/Forces and Moments/Landing_Gear/LG Friction new ==
  data: roll_f input; HaG input; rigidbodyBus input; nws input; force_other input; torque_other input; force_b output; torque_b output; vehicle parameter; stepsize_fm parameter
function [force_b,torque_b] = landing_gear_friction(roll_f,HaG,rigidbodyBus,nws,force_other,torque_other,vehicle,stepsize_fm)
%constants
reduced_fric_nw = 0.2; %reduced friction at aux wheel when turning

% variables
euler = rigidbodyBus.euler;
Vg = rigidbodyBus.Vg;
omega = rigidbodyBus.omega;

%trafos
Tfg = angle2rotation(euler(1),euler(2),euler(3)); % Tfg => transformation matrix geodetic to body
Tgf = Tfg';                                       % Tgf => transformation matrix body to geodetic
Tfl = angle2rotation(euler(1),euler(2),0);        % Tfl => transformation matrix flat x-y to body
Tlf = Tfl';
Tlg = Tlf*Tfg;                                    % Tlg => transformation matrix geodetic to flat x-y
Tgl = Tlg';
Tlw = angle2rotation(0,0,nws);                    % Tlw => transformation matrix nose/tail wheel to flat x-y
Twl = Tlw';
Tfw = Tfl*Tlw;                                    % Tfw => transformation matrix nose/tail wheel to body
Twf = Tfw';

%% calculate compression
gear = vehicle.gear;
CG   = vehicle.cg;
m    = vehicle.m;

pos_right_cg = gear.right_pos - CG;
pos_left_cg  = gear.left_pos - CG;
pos_aux_cg  = gear.aux_pos - CG;

pos_right_g = Tgf * pos_right_cg;
pos_left_g  = Tgf * pos_left_cg;
pos_aux_g  = Tgf * pos_aux_cg;

pos_right_l = Tlf * pos_right_cg;
pos_left_l  = Tlf * pos_left_cg;
pos_aux_l  = Tlf * pos_aux_cg;

compression_right = max(0,pos_right_g(3) - HaG);
compression_left  = max(0,pos_left_g(3)  - HaG);
compression_aux  = max(0,pos_aux_g(3)  - HaG);

%% gear friction
force_other_flat  = Tlf * force_other;
% force_other_wheel  = Twf * force_other;
torque_other_flat = Tlf * torque_other;

LG_force = single([0;0;0]);
LG_torque = single([0;0;0]);

rWoW = compression_right > 0;
lWoW = compression_left > 0;
aWoW = compression_aux > 0;

num_wheels = single(aWoW+rWoW+lWoW);

if rWoW || lWoW
    % main wheels touch ground
    Vl = Tlg*Vg; %velocity in x_y plane aligned to aircraft orientation
    omegaL = Tlf * omega;
    Vl_right = Vl + cross(omegaL, pos_right_l); %right wheel velocity
    Vl_left = Vl + cross(omegaL, pos_left_l); %left wheel velocity

    % lateral forces
    force_lat_opp = force_other_flat(2) + (single(rWoW) + single(lWoW))/2 * Vl(2)*m/stepsize_fm; %other lateral forces (in opposite
    force_lat = -force_lat_opp;
    LG_force = LG_force + [0; force_lat; 0];

    % longitudinal forces
    force_lon_opp_right = force_other_flat(1)/num_wheels + Vl_right(1)*m/stepsize_fm/num_wheels; %opposing forces
    force_lon_opp_left = force_other_flat(1)/num_wheels + Vl_left(1)*m/stepsize_fm/num_wheels; %opposing forces
    force_lon_right = -sign(force_lon_opp_right) * single(rWoW) * min(roll_f/num_wheels, abs(force_lon_opp_right));
    force_lon_left = -sign(force_lon_opp_left) * single(lWoW) * min(roll_f/num_wheels, abs(force_lon_opp_left));
    LG_force = LG_force + [force_lon_right + force_lon_left; 0; 0];
end
if aWoW
    % aux wheel also touches ground
    LG_torque = LG_torque + [0; 0; -torque_other_flat(3)]; % compensate all yaw torques

    Vw = Twl*Tlg*Vg; %velocity in x_y plane aligned to nose/tail wheel orientation
    omegaW = Twf * omega;
    Vw_aux = Vw + cross(omegaW, pos_aux_l); %nose/tail wheel velocity
    % lateral forces
    force_lat_opp = Vw_aux(2)*m/stepsize_fm * reduced_fric_nw; %other lateral forces (in opposite
    force_lat = Tlw * [0;force_lat_opp;0];
    LG_force = LG_force + [0; force_lat(2); 0]; %in flat coordinates
    %longitudinal forces
    force_lon_opp = Vw_aux(1)*m/stepsize_fm/num_wheels; %opposing forces
    force_lon = -sign(force_lon_opp) * min(roll_f/num_wheels, abs(force_lon_opp));
    LG_force = LG_force + [force_lon; 0; 0]; %in flat coordinates
    %yaw torques
    r_torque = -pos_aux_l(1) * force_lat(2);
    LG_torque = LG_torque + [0; 0; r_torque];
end

force_g   = Tgl * LG_force;
torque_g  = Tgl * LG_torque;

force_b   = Tfg * force_g;
torque_b  = Tfg * torque_g;

end

function dcm = angle2rotation(phi,theta,psi)
t1 = [1 0 0;0 cos(phi) sin(phi);0 -sin(phi) cos(phi)];
t2 = [cos(theta) 0 -sin(theta);0 1 0;sin(theta) 0 cos(theta)];
t3 = [cos(psi) sin(psi) 0;-sin(psi) cos(psi) 0;0 0 1];
dcm = t1*t2*t3;
end

== matlab function fm_gram/Actuator Model/Servos ==
  data: ail input; ele input; rud input; thr input; ail_cmd input; ele_cmd input; rud_cmd input; dail output; dele output; drud output; dthr output; thr_cmd input; servo parameter
function [dail,dele,drud,dthr]= servos(ail,ele,rud,thr,ail_cmd,ele_cmd,rud_cmd,thr_cmd,servo)
T_ail = servo.T(1);
T_ele = servo.T(2);
T_rud = servo.T(3);
T_thr = servo.T(4);

dail = 1/T_ail*(ail_cmd*servo.pwmToAngle(1)-ail);
dele = 1/T_ele*(ele_cmd*servo.pwmToAngle(2)-ele);
drud = 1/T_rud*(rud_cmd*servo.pwmToAngle(3)-rud);
dthr = 1/T_thr*(thr_cmd-thr);

end
